simulink model "p6simulink"  (R2025b)
settings: Solver=VariableStepAuto  StartTime=0.0  StopTime=0.005  RelTol=1e-3
settings Model: Creator=raul  LastModifiedBy=raul

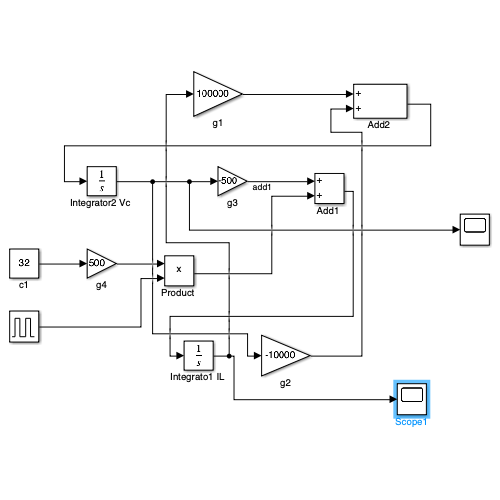
[thumbnail: Simulink's stored preview of the top-level diagram]
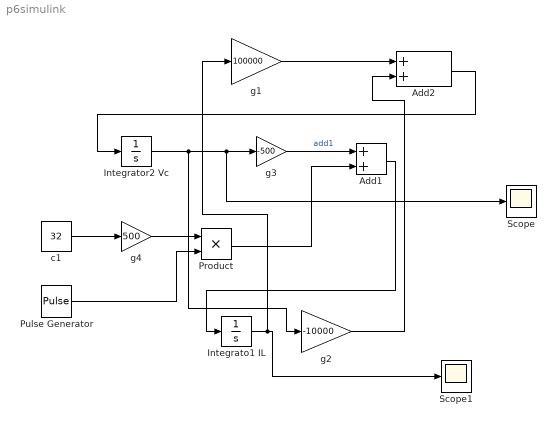
== system p6simulink ==
  "Add1 " : Sum
  "Add2 " : Sum
  "Integrato1 IL " : Integrator
  "Integrator2 Vc " : Integrator
  "Product " : Product
  Pulse Generator : DiscretePulseGenerator  PulseType=Time based  Period=1e-5  PulseWidth=40
  Scope : Scope
      settings: ActiveDisplayYMinimum=-1.6690763206549946  ActiveDisplayYMaximum=15.021686885894955
  Scope1 : Scope
      settings: ActiveDisplayYMinimum=-0.17312047082165338  ActiveDisplayYMaximum=1.5580842373948807
  c1 : Constant  Value=32
  g1 : Gain  Gain=100000
  g2 : Gain  Gain=-10000
  g3 : Gain  Gain=-500
  g4 : Gain  Gain=500
  wires:
  c1/1 -> g4/1
  g4/1 -> "Product "/1
  Pulse Generator/1 -> "Product "/2
  "Integrator2 Vc "/1 -> g2/1, Scope/1, g3/1
  "Product "/1 -> "Add1 "/2
  g3/1 -> "Add1 "/1  "add1"
  g1/1 -> "Add2 "/1
  "Integrato1 IL "/1 -> g1/1, Scope1/1
  "Add1 "/1 -> "Integrato1 IL "/1
  "Add2 "/1 -> "Integrator2 Vc "/1
  g2/1 -> "Add2 "/2
